simulink model "gm_bch_encoder_model"  (R2020b)
settings: Solver=FixedStepDiscrete  StartTime=0.0  StopTime=2  RelTol=1e-3
undefined symbols (not defined in the file or in its folder): lfsr_message
libraries: simulink x1, whdlio x1, hdlsllib x1
settings Model: Creator=EFlores  LastModifiedBy=wardo
settings SolverCC: AutoInsertRateTranBlk=on
settings DataIOCC: LimitDataPoints=on  SaveOutput=off  SaveTime=off
settings OptimizationCC: BlockReduction=off  ConditionallyExecuteInputs=off  DefaultParameterBehavior=Inlined  LifeSpan=inf
settings DebuggingCC: AlgebraicLoopMsg=error  InheritedTsInSrcMsg=none  SingleTaskRateTransMsg=error  AllowSymbolicDim=off  StrictBusMsg=ErrorOnBusTreatedAsVector  SFUnexpectedBacktrackingDiag=warning  SFNoUnconditionalDefaultTransitionDiag=warning  SFExecutionAtInitializationDiag=none  ArithmeticOperatorsInVariantConditions=warning
settings HardwareCC: ProdBitPerPointer=32  ProdBitPerSizeT=32  ProdBitPerPtrDiffT=32  ProdLargestAtomicFloat=None  ProdIntDivRoundTo=Undefined  ProdEndianess=Unspecified  ProdWordSize=32  ProdHWDeviceType=ASIC/FPGA->ASIC/FPGA  ProdEqTarget=off
settings SFSimCC: SimUseLocalCustomCode=off  CustomCodeUndefinedFunction=UseInterfaceOnly
settings RTWCC: RTWUseLocalCustomCode=off
settings CodeAppCC: StateflowObjectComments=on
settings GRTTargetCC: TargetLangStandard=C89/C90 (ANSI)
settings ConfigComp: CovScope=ReferencedModels  CovMetricSettings=dw  CovSaveCumulativeToWorkspaceVar=on  CovSaveSingleToWorkspaceVar=on  CovExternalEMLEnable=off  CovSFcnEnable=off

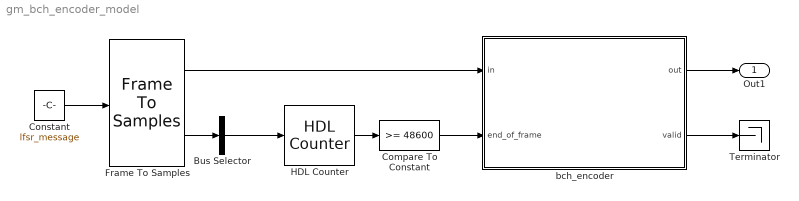
== system gm_bch_encoder_model ==
  Bus Selector : BusSelector  OutputSignals=valid
  Compare To Constant : simulink/Logic and Bit Operations/Compare To Constant  relop=>=  const=48600  OutDataTypeStr=boolean
  Constant : Constant  Value=lfsr_message  OutDataTypeStr=fixdt(0,1,0)  SampleTime=1
  Frame To Samples : whdlio/Frame To Samples  InterSampleIdleCycles=0  InterFrameIdleCycles=0  OutputSize=1  InterleaveSamples=off
      settings: SourceProductBaseCode=LH
  HDL Counter : hdlsllib/Sources/HDL Counter  CountType=Count limited  CountInit=1  CountStep=1  CountMax=48600  CountFromType=Initial value  CountFrom=1  CountResetPort=off  CountLoadPort=off  CountEnbPort=on  CountDirPort=off  CountDataType=Unsigned  CountWordLen=16  CountFracLen=0  CountSampTime=1
  Terminator : Terminator
  bch_encoder : Subsystem
  Out1 : Outport  VectorParamsAs1DForOutWhenUnconnected=off
  wires:
  bch_encoder/2(valid) -> Terminator/1
  Compare To Constant/1 -> bch_encoder/2(end_of_frame)
  HDL Counter/1 -> Compare To Constant/1
  Bus Selector/1 -> HDL Counter/1
  Frame To Samples/2 -> Bus Selector/1
  Constant/1 -> Frame To Samples/1
  bch_encoder/1(out) -> Out1/1
  Frame To Samples/1 -> bch_encoder/1(in)

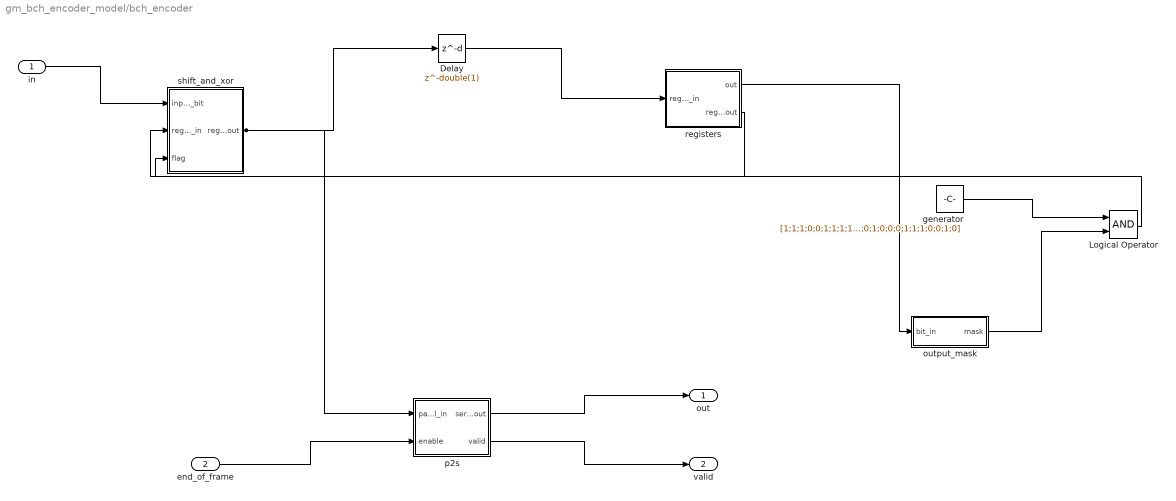
== system gm_bch_encoder_model/bch_encoder ==
  in : Inport  OutDataTypeStr=fixdt(0, 1, 0)  PortDimensions=1  SampleTime=2.05761316872428e-05
  end_of_frame : Inport  Port=2  OutDataTypeStr=boolean  PortDimensions=1  SampleTime=2.05761316872428e-05
  Delay : Delay  DelayLength=double(1)  InitialCondition=0  SampleTime=2.05761316872428e-05
  Logical Operator : Logic  AllPortsSameDT=off  OutDataTypeStr=fixdt(0, 1, 0)  SampleTime=2.05761316872428e-05
  generator : Constant  Value=[1;1;1;0;0;1;1;1;1;0;1;0;1;0;1;0;0;1;0;0;0;0;0;0;0;1;1;0;0;1;1;0;1;1;1;0;1;1;1;1;1;0;1;0;0;0;0;1;1;1;1;0;0;0;1;0;1;1;0;0;0;0;0;0;1;0;0;1;0;0;0;1;0;0;0;1;0;0;0;0;1;0;1;0;1;1;0;0;0;0;1;1;1;0;1;1;0;0;0;1;1;0;1;1;0;0;1;1;0;1;0;0;1;1;1;1;0;0;1;1;0;0;0;0;1;0;1;0;0;0;1;1;1;0;0;0;1;0;0;0;1;0;1;0;0;0;1;1;1;0;1;0;0;0;1;0;0;0;0;1;1;1;0;0;0;0;0;1;0;1;1;1;0;0;0;0;0;1;1;0;0;1;0;0;0;1;1;1;0;0;1;0]  OutDataTypeStr=fixdt(0, 1, 0)  SampleTime=2.05761316872428e-05
  output_mask : Subsystem
  p2s : Subsystem
  registers : Subsystem
  shift_and_xor : Subsystem
  out : Outport  VectorParamsAs1DForOutWhenUnconnected=off
  valid : Outport  Port=2  VectorParamsAs1DForOutWhenUnconnected=off
  wires:
  in/1 -> shift_and_xor/1(input_bit)
  end_of_frame/1 -> p2s/2(enable)
  Delay/1 -> registers/1(registers_in)
  Logical Operator/1 -> shift_and_xor/3(flag)
  generator/1 -> Logical Operator/1
  output_mask/1(mask) -> Logical Operator/2
  p2s/1(serial_out) -> out/1
  p2s/2(valid) -> valid/1
  registers/1(out) -> output_mask/1(bit_in)
  registers/2(registers_out) -> shift_and_xor/2(registers_in)
  shift_and_xor/1(registers_out) -> Delay/1, p2s/1(parallel_in)

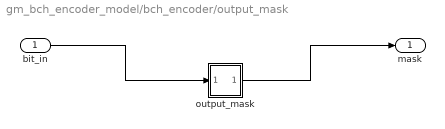
== system gm_bch_encoder_model/bch_encoder/output_mask ==
  bit_in : Inport  OutDataTypeStr=fixdt(0, 1, 0)  PortDimensions=1  SampleTime=2.05761316872428e-05
  output_mask : MATLAB Function  TreatAsAtomicUnit=on
  mask : Outport  VectorParamsAs1DForOutWhenUnconnected=off
  wires:
  bit_in/1 -> output_mask/1(bit_in)
  output_mask/1(mask) -> mask/1

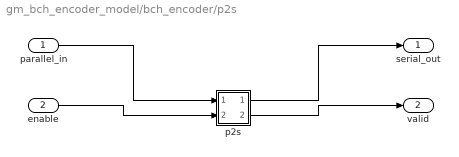
== system gm_bch_encoder_model/bch_encoder/p2s ==
  parallel_in : Inport  OutDataTypeStr=fixdt(0, 1, 0)  PortDimensions=[192]  SampleTime=2.05761316872428e-05
  enable : Inport  Port=2  OutDataTypeStr=boolean  PortDimensions=1  SampleTime=2.05761316872428e-05
  p2s : MATLAB Function  TreatAsAtomicUnit=on  mask{input_length=192}
  serial_out : Outport  VectorParamsAs1DForOutWhenUnconnected=off
  valid : Outport  Port=2
  wires:
  parallel_in/1 -> p2s/1(parallel_in)
  enable/1 -> p2s/2(enable)
  p2s/1(serial_out) -> serial_out/1
  p2s/2(valid) -> valid/1

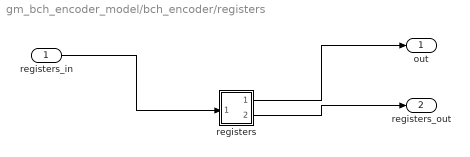
== system gm_bch_encoder_model/bch_encoder/registers ==
  registers_in : Inport  OutDataTypeStr=fixdt(0, 1, 0)  PortDimensions=[192]  SampleTime=2.05761316872428e-05
  registers : MATLAB Function  TreatAsAtomicUnit=on
  out : Outport  VectorParamsAs1DForOutWhenUnconnected=off
  registers_out : Outport  Port=2
  wires:
  registers_in/1 -> registers/1(registers_in)
  registers/1(out) -> out/1
  registers/2(registers_out) -> registers_out/1

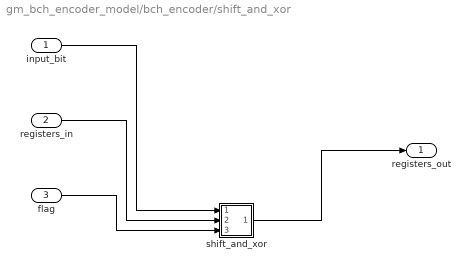
== system gm_bch_encoder_model/bch_encoder/shift_and_xor ==
  input_bit : Inport  OutDataTypeStr=fixdt(0, 1, 0)  PortDimensions=1  SampleTime=2.05761316872428e-05
  registers_in : Inport  Port=2  OutDataTypeStr=fixdt(0, 1, 0)  PortDimensions=[192]  SampleTime=2.05761316872428e-05
  flag : Inport  Port=3  OutDataTypeStr=fixdt(0, 1, 0)  PortDimensions=[192]  SampleTime=2.05761316872428e-05
  shift_and_xor : MATLAB Function  TreatAsAtomicUnit=on
  registers_out : Outport  VectorParamsAs1DForOutWhenUnconnected=off
  wires:
  input_bit/1 -> shift_and_xor/1(input_bit)
  registers_in/1 -> shift_and_xor/2(registers_in)
  flag/1 -> shift_and_xor/3(flag)
  shift_and_xor/1(registers_out) -> registers_out/1

== matlab function gm_bch_encoder_model/bch_encoder/registers/registers ==
  settings: fimath=fimath('RoundingMethod', 'Floor','OverflowAction', 'Wrap','ProductMode', 'FullPrecision', 'SumMode', 'FullPrecision')
  data: registers_in input; out output fixdt(0,1,0) size=1; registers_out output fixdt(0,1,0) size=192
function [out, registers_out] = state_registers(registers_in)
%#codegen

persistent lfsr;
if isempty(lfsr)
    lfsr = fi(zeros(192, 1), 0, 1, 0);
else
    lfsr = registers_in;
end
out = lfsr(192);
registers_out = lfsr;

== matlab function gm_bch_encoder_model/bch_encoder/output_mask/output_mask ==
  settings: fimath=fimath('RoundingMethod', 'Floor','OverflowAction', 'Wrap','ProductMode', 'FullPrecision', 'SumMode', 'FullPrecision')
  data: bit_in input; mask output
function mask = bitmask(bit_in)
%#codegen

if bit_in
    mask = fi(ones(192, 1), 0, 1, 0);
else
    mask = fi(zeros(192, 1), 0, 1, 0);
end

== matlab function gm_bch_encoder_model/bch_encoder/shift_and_xor/shift_and_xor ==
  settings: fimath=fimath('RoundingMethod', 'Floor','OverflowAction', 'Wrap','ProductMode', 'FullPrecision', 'SumMode', 'FullPrecision')
  data: input_bit input; registers_out output fixdt(0,1,0); registers_in input; flag input
function registers_out = shift_and_xor(input_bit, registers_in, flag)
%#codegen
buffer = [input_bit; registers_in(1:192-1)];
registers_out = fi(xor(buffer, flag), 0, 1, 0);

== matlab function gm_bch_encoder_model/bch_encoder/p2s/p2s ==
  settings: fimath=fimath('RoundingMethod', 'Floor','OverflowAction', 'Wrap','ProductMode', 'FullPrecision', 'SumMode', 'FullPrecision')
  data: parallel_in input; serial_out output fixdt(0,1,0); enable input; input_length parameter uint16; valid output
function [serial_out, valid] = p2s_buffer(parallel_in, enable, input_length)
%#codegen

state_iddle    = 0;
state_reading  = 1;

persistent moore_state_machine;
if isempty(moore_state_machine)
    moore_state_machine = fi(0, 0, 1, 0);
end

persistent counter;
if isempty(counter)
    counter = fi(1, 0, 16, 0);
end

persistent buffer;
if isempty(buffer)
    buffer = parallel_in;
end

switch moore_state_machine
    case state_iddle
        serial_out = fi(0, 0, 1, 0);
        valid      = fi(0, 0, 1, 0);
        if enable
            moore_state_machine(1) = state_reading;
            buffer = parallel_in;
            serial_out          = buffer(input_length+1-counter);
            valid      = fi(1, 0, 1, 0);
            counter             = fi(counter + 1, 0, 16, 0);
        end
    case state_reading
        serial_out = buffer(input_length+1-counter);
        counter    = fi(counter + 1, 0, 16, 0);
        valid      = fi(1, 0, 1, 0);
        if(counter > input_length)
            counter = fi(1, 0, 16, 0);
            moore_state_machine(1) = state_iddle;
        end
    otherwise
        serial_out = fi(0, 0, 1, 0);
        valid      = fi(0, 0, 1, 0);
end
